simulink model "equazione"  (R2017a)
settings: Solver=VariableStepAuto  StartTime=k*Tc  StopTime=(k+1)*Tc  RelTol=1e-3
settings Model: Creator=Enrico Donato  LastModifiedBy=Enrico Donato
settings DataIOCC: LoadExternalInput=on  LoadInitialState=on  SaveFinalState=on  SaveFormat=Array  SaveState=on

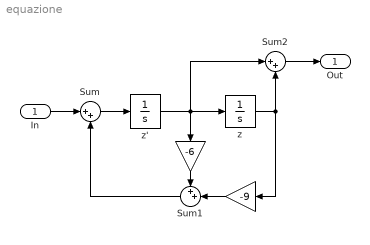
== system equazione ==
  In : Inport
  " " : Gain  Gain=-6
  " " : Gain  Gain=-9
  Sum : Sum  Inputs=|++
  Sum1 : Sum  Inputs=++|
  Sum2 : Sum  Inputs=|++
  z : Integrator
  z' : Integrator
  Out : Outport
  wires:
  z'/1 -> " "/1, z/1, Sum2/1
  z/1 -> " "/1, Sum2/2
  Sum/1 -> z'/1
  Sum1/1 -> Sum/2
  " "/1 -> Sum1/2
  " "/1 -> Sum1/1
  Sum2/1 -> Out/1
  In/1 -> Sum/1
